simulink model "AUV_SLIDDING_OPTIMAL_2"  (Simulink 7.6)
settings: Solver=ode5  StartTime=0.0  StopTime=200  FixedStep=.1  RelTol=1e-3
libraries: simulink x3
settings Model: Creator=Comp  LastModifiedBy=HP

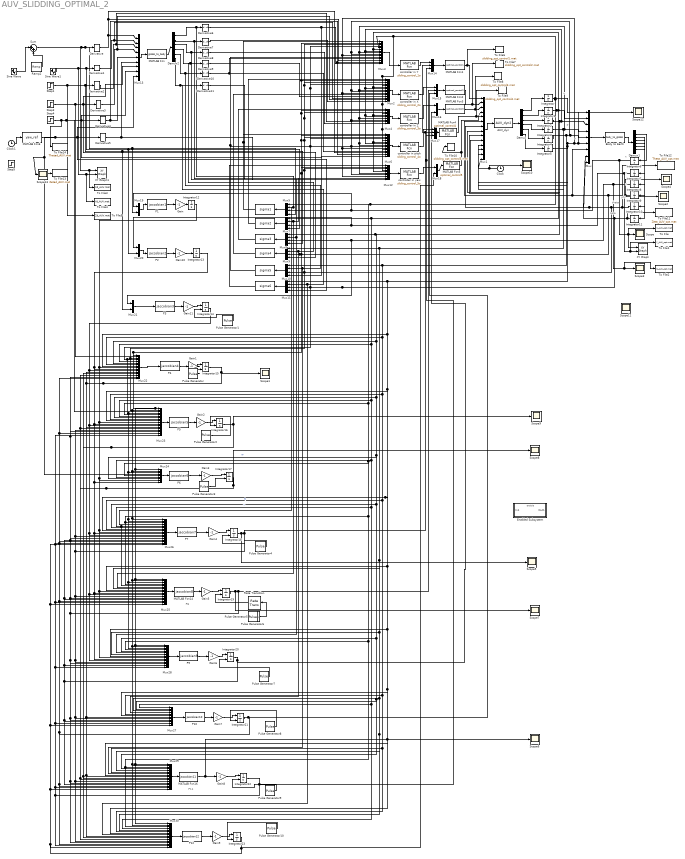
== system AUV_SLIDDING_OPTIMAL_2 ==
  note: u
  note: p
  note: r
  note: x
  note: y
  note: z
  note: phi
  note: theta
  note: zeta
  note: P8
  note: P11
  " " : MATLABFcn  MATLABFcn=sigma6
  "   " : MATLABFcn  MATLABFcn=sigma5
  "    " : MATLABFcn  MATLABFcn=sigma4
  "      " : MATLABFcn  MATLABFcn=sigma3
  "            " : MATLABFcn  MATLABFcn=sigma2
  "                            " : MATLABFcn  MATLABFcn=sigma1
  AUV_dyn : MATLABFcn  MATLABFcn=AUV_dyn2
  Body to Earth : MATLABFcn  MATLABFcn=body_to_global
  Clock : Clock
      settings: Decimation=10
  Clock1 : Clock
  Demux : Demux  Outputs=6
  Demux1 : Demux  Outputs=6
  Demux2 : Demux  Outputs=6
  Derivative{,1..11} (12 alike) : Derivative
  Enabled Subsystem : Subsystem  TreatAsAtomicUnit=on
  Gain{,1..11} (12 alike) : Gain  Gain=-1
  Integrator{,1..6,8..13} (13 alike) : Integrator
  Integrator{14..23} (10 alike) : Integrator  ExternalReset=rising
  Integrator7 : Integrator  InitialCondition=12.5
  MATLAB Fcn : MATLABFcn  MATLABFcn=global_to_body
  MATLAB Fcn1 : MATLABFcn  MATLABFcn=optimal_control1
  MATLAB Fcn14 : MATLABFcn  MATLABFcn=jaccobian8
  MATLAB Fcn16 : MATLABFcn  MATLABFcn=jaccobian11
  MATLAB Fcn2 : MATLABFcn  MATLABFcn=optimal_control2
  MATLAB Fcn3 : MATLABFcn  MATLABFcn=optimal_control3
  MATLAB Fcn4 : MATLABFcn  MATLABFcn=optimal_control4
  MATLAB Fcn5 : MATLABFcn  MATLABFcn=optimal_control5
  MATLAB Fcn6 : MATLABFcn  MATLABFcn=yaw_ref
  Mux : Mux  Inputs=9
  Mux1 : Mux  Inputs=14
  Mux{5,7..11} (6 alike) : Mux
  Mux12 : Mux  Inputs=10
  Mux13 : Mux  Inputs=9
  Mux14 : Mux  Inputs=3
  Mux15 : Mux  Inputs=3
  Mux{16,18..21} (5 alike) : Mux  Inputs=2
  Mux17 : Mux  Inputs=3
  Mux{2..3,6,28} (4 alike) : Mux  Inputs=15
  Mux22 : Mux  Inputs=16
  Mux23 : Mux  Inputs=18
  Mux24 : Mux  Inputs=9
  Mux25 : Mux  Inputs=17
  Mux26 : Mux  Inputs=17
  Mux27 : Mux  Inputs=12
  Mux29 : Mux  Inputs=17
  Mux30 : Mux  Inputs=16
  Mux4 : Mux  Inputs=10
  P1 : MATLABFcn  MATLABFcn=jaccobian1
  P10 : MATLABFcn  MATLABFcn=jaccobian10
  P12 : MATLABFcn  MATLABFcn=jaccobian12
  P2 : MATLABFcn  MATLABFcn=jaccobian2
  P3 : MATLABFcn  MATLABFcn=jaccobian3
  P4 : MATLABFcn  MATLABFcn=jaccobian4
  P5 : MATLABFcn  MATLABFcn=jaccobian5
  P6 : MATLABFcn  MATLABFcn=jaccobian6
  P7 : MATLABFcn  MATLABFcn=jaccobian7
  P9 : MATLABFcn  MATLABFcn=jaccobian9
  Pulse Generator{,1..5,7..10} (10 alike) : DiscretePulseGenerator  PulseType=Time based  Period=1  PulseWidth=50
  Pulse Generator6 : DiscretePulseGenerator
  Ramp2 : simulink/Sources/Ramp  SystemSampleTime=-1  slope=.25  start=0  X0=0
  Rate Transition : RateTransition
  Scope{,1..13} (14 alike) : Scope
      Scope1 settings: YMin=-2e+007  YMax=1.8e+008
      Scope10 settings: YMin=0  YMax=160  SaveName=ScopeData10
      Scope11 settings: SaveName=ScopeData11
      Scope12 settings: YMin=-0.05  YMax=0.6  SaveName=ScopeData12
      Scope13 settings: YMin=0  YMax=250  SaveName=ScopeData13
      Scope2 settings: YMin=-0.08  YMax=0.01  SaveName=ScopeData2
      Scope3 settings: SaveName=ScopeData3
      Scope4 settings: YMin=1  YMax=8.5  SaveName=ScopeData4
      Scope5 settings: YMin=0  YMax=250  SaveName=ScopeData5
      Scope6 settings: SaveName=ScopeData6
      Scope7 settings: YMin=-4.5e+008  YMax=4.5e+008  SaveName=ScopeData7
      Scope8 settings: YMin=-1000  YMax=1750  SaveName=ScopeData8
      Scope9 settings: YMin=-4e+006  YMax=7.5e+006  SaveName=ScopeData9
  Sine Wave : Sin  Amplitude=2.5  Frequency=.1  SampleTime=0
  Sine Wave1 : Sin  Amplitude=12.5  Frequency=.05  Phase=pi/2  SampleTime=0
  Step1 : Step  Time=0  After=5  SampleTime=0
  Step3 : Step  Time=0  After=0  SampleTime=0
  Step4 : Step  Time=0  After=0  SampleTime=0
  Step5 : Step  Time=0  After=0  SampleTime=0
  Sum : Sum  Inputs=|++
  To File : ToFile  Filename=X_AUV_opt.mat  MatrixName=Xo  SaveFormat=Timeseries
  To File1 : ToFile  Filename=Y_AUV_opt.mat  MatrixName=Yo  SaveFormat=Timeseries
  To File10 : ToFile  Filename=slidding_opt_control5.mat  MatrixName=Uo5  SaveFormat=Timeseries
  To File11 : ToFile  Filename=Zeta_AUV_opt.mat  MatrixName=zeta_o  SaveFormat=Timeseries
  To File12 : ToFile  Filename=Theta_AUV_opt.mat  MatrixName=theta_o  SaveFormat=Timeseries
  To File13 : ToFile  Filename=Zetad_AUV.mat  MatrixName=zeta_d  SaveFormat=Timeseries
  To File14 : ToFile  Filename=Thetad_AUV.mat  MatrixName=theta_d  SaveFormat=Timeseries
  To File2 : ToFile  Filename=Z_AUV_opt.mat  MatrixName=Zo  SaveFormat=Timeseries
  To File3 : ToFile  Filename=Xd_AUV.mat  MatrixName=Xd  SaveFormat=Timeseries
  To File4 : ToFile  Filename=Yd_AUV.mat  MatrixName=Yd  SaveFormat=Timeseries
  To File5 : ToFile  Filename=Zd_AUV.mat  MatrixName=Zd  SaveFormat=Timeseries
  To File6 : ToFile  Filename=slidding_opt_control1.mat  MatrixName=Uo1  SaveFormat=Timeseries
  To File7 : ToFile  Filename=slidding_opt_control2.mat  MatrixName=Uo2  SaveFormat=Timeseries
  To File8 : ToFile  Filename=slidding_opt_control3.mat  MatrixName=Uo3  SaveFormat=Timeseries
  To File9 : ToFile  Filename=slidding_opt_control4.mat  MatrixName=Uo4  SaveFormat=Timeseries
  XY Graph : simulink/Sinks/XY Graph  SystemSampleTime=-1  xmin=0  xmax=60  ymin=-20  ymax=20  st=-1
  XY Graph1 : simulink/Sinks/XY Graph  SystemSampleTime=-1  xmin=-20  xmax=20  ymin=-20  ymax=20  st=-1
  controller in X : MATLABFcn  MATLABFcn=sliding_control_2o
  controller in Y : MATLABFcn  MATLABFcn=sliding_control_1o
  controller in Z : MATLABFcn  MATLABFcn=sliding_control_3o
  controller in pitch : MATLABFcn  MATLABFcn=sliding_control_4o
  controller in yaw : MATLABFcn  MATLABFcn=sliding_control_5o
  wires:
  AUV_dyn/1 -> Demux/1
  Demux/1 -> Integrator/1
  Demux/2 -> Integrator1/1
  Demux/3 -> Integrator2/1
  Demux/4 -> Integrator3/1
  Demux/5 -> Integrator4/1
  Demux/6 -> Integrator5/1
  Integrator2/1 -> Mux1/10, Mux/3, Mux3/7, Mux2/7, Mux4/6, Mux6/7, Mux8/1, Mux22/6, Mux23/7, Mux24/7, Mux26/6, Mux28/5, Mux27/2, Mux29/4  "w"
  Integrator4/1 -> Mux1/12, Mux/5, Mux3/9, Mux2/9, Mux4/8, Mux6/9, Mux12/7, Mux10/1, Mux22/7, Mux23/8, Mux26/7, Mux27/5, Mux29/6, Mux30/6  "q"
  Integrator3/1 -> Mux1/11, Mux/4, Mux3/8, Mux2/8, Mux4/7, Mux6/8, Mux12/6, Mux9/1, Mux25/7, Mux28/7, Mux27/3, Mux29/5, Mux30/5
  Mux/1 -> Body to Earth/1
  Integrator/1 -> Mux/1, Mux1/8, Mux3/5, Mux2/5, Mux4/4, Mux6/5, Mux12/4, Mux5/1, Mux23/5, Mux24/5, Mux26/3, Mux25/4, Mux28/4, Mux29/3, Mux30/3
  Integrator1/1 -> Mux/2, Mux1/9, Mux3/6, Mux2/6, Mux4/5, Mux6/6, Mux12/5, Mux7/1, Mux22/5, Mux23/6, Mux24/6, Mux26/5, Mux25/5, Mux27/1, Mux30/4  "v"
  Integrator5/1 -> Mux1/13, Mux3/10, Mux2/10, Mux6/10, Mux12/8, Mux/6, Scope12/1, Mux11/1, Mux22/8, Mux23/9, Mux26/8, Mux25/8, Mux28/8, Mux27/6, Mux29/8, Mux30/7
  Body to Earth/1 -> Demux1/1
  Demux1/1 -> Integrator6/1
  Demux1/2 -> Integrator7/1
  Demux1/3 -> Integrator8/1
  Demux1/4 -> Integrator9/1
  Demux1/5 -> Integrator10/1
  Demux1/6 -> Integrator11/1
  Integrator9/1 -> Mux/7, Mux1/6, Mux3/2, Mux2/2, Mux4/2, Mux6/2, Mux12/2, Mux9/3, Mux22/1, Mux23/1, Mux24/1, Mux25/1, Mux28/1, Mux29/1, Mux30/1, Scope4/1, Scope2/1
  Integrator10/1 -> Mux/8, Mux1/7, Mux10/3, Mux3/3, Mux2/3, Mux4/3, Mux6/3, Mux12/3, Mux22/3, Mux23/2, Mux24/2, Mux26/1, Mux25/2, Mux28/2, Mux29/2, Mux30/2, To File12/1
  Integrator11/1 -> Mux/9, Mux11/3, Mux3/4, Mux2/4, Mux6/4, Mux22/4, Mux23/4, Mux24/3, Mux26/2, Mux25/3, Mux28/3, To File11/1
  Mux5/1 -> "                            "/1
  Integrator6/1 -> Scope/1, XY Graph/1, To File/1, Mux5/3, Mux19/1
  Mux7/1 -> "            "/1
  Integrator7/1 -> XY Graph/2, To File1/1, Mux7/3, Mux20/1
  Mux8/1 -> "      "/1
  Integrator8/1 -> Mux8/3, Mux21/1, Scope3/1, To File2/1
  Mux9/1 -> "    "/1
  Mux10/1 -> "   "/1
  Mux11/1 -> " "/1
  Mux3/1 -> controller in Y/1
  "                            "/1 -> Mux3/1, Mux6/1
  Mux2/1 -> controller in X/1
  Mux4/1 -> controller in Z/1
  Mux6/1 -> controller in pitch/1
  Mux12/1 -> controller in yaw/1
  "   "/1 -> Mux3/11, Mux6/11
  "            "/1 -> Mux2/1
  "    "/1 -> Mux2/11
  "      "/1 -> Mux4/1
  " "/1 -> Mux12/1
  Sum/1 -> Derivative/1, Mux5/4, Mux19/2, XY Graph1/1, To File3/1
  Sine Wave1/1 -> Derivative1/1, Mux7/4, Mux20/2, XY Graph1/2, To File4/1
  Step1/1 -> Derivative2/1, Mux8/4, Mux21/2, To File5/1
  Step3/1 -> Derivative3/1, Mux13/7, Mux9/4, Mux22/2
  Step4/1 -> Derivative4/1, Mux13/8, Mux10/4, Mux23/3, To File14/1
  MATLAB Fcn6/1 -> Derivative5/1, Mux13/9, Mux11/4, Mux24/4, To File13/1, Scope13/1
  Derivative/1 -> Mux13/1, Mux3/13, Mux6/13
  Derivative1/1 -> Mux13/2, Mux2/13
  Derivative2/1 -> Mux13/3, Mux4/9
  Derivative3/1 -> Mux13/4, Mux2/14
  Derivative4/1 -> Mux13/5, Mux3/14, Mux6/14
  Derivative5/1 -> Mux13/6, Mux12/10
  Mux13/1 -> MATLAB Fcn/1
  Demux2/1 -> Derivative6/1, Mux5/2, Mux26/4
  Demux2/2 -> Derivative7/1, Mux7/2, Mux25/6
  Demux2/3 -> Derivative8/1, Mux8/2, Mux28/6
  Demux2/4 -> Derivative9/1, Mux9/2, Mux27/4
  Demux2/5 -> Derivative10/1, Mux10/2, Mux29/7
  Demux2/6 -> Derivative11/1, Mux11/2, Mux30/8
  Derivative10/1 -> Mux3/12, Mux6/12
  Derivative6/1 -> Mux3/15, Mux6/15
  Derivative9/1 -> Mux2/12
  Derivative7/1 -> Mux2/15
  Derivative8/1 -> Mux4/10
  Derivative11/1 -> Mux12/9
  MATLAB Fcn/1 -> Demux2/1
  MATLAB Fcn1/1 -> Mux1/1, To File6/1
  controller in Y/1 -> Mux14/1
  Mux14/1 -> MATLAB Fcn1/1
  Mux15/1 -> MATLAB Fcn2/1
  MATLAB Fcn2/1 -> Mux1/2, To File7/1
  controller in X/1 -> Mux15/1
  Mux16/1 -> MATLAB Fcn3/1
  MATLAB Fcn3/1 -> Mux1/3, To File8/1
  controller in Z/1 -> Mux16/1
  MATLAB Fcn4/1 -> Mux1/4, To File9/1
  Mux17/1 -> MATLAB Fcn4/1
  controller in pitch/1 -> Mux17/1
  MATLAB Fcn5/1 -> Mux1/5, To File10/1
  Mux18/1 -> MATLAB Fcn5/1
  controller in yaw/1 -> Mux18/1
  Mux19/1 -> P1/1
  Mux20/1 -> P2/1
  Mux21/1 -> P3/1
  Mux22/1 -> P4/1
  Integrator12/1 -> Mux22/9, Mux23/10, Mux24/8, Mux26/9, Mux25/9, Mux28/9
  Integrator13/1 -> Mux22/10, Mux23/11, Mux24/9, Mux26/10, Mux25/10, Mux28/10
  Integrator14/1 -> Mux22/11, Mux23/12, Mux26/11, Mux25/11, Mux28/11
  Integrator15/1 -> Mux22/12, Mux23/13, Mux27/7, Mux29/9, Mux30/9, Scope1/1
  Integrator16/1 -> Mux22/13, Mux29/10, Mux30/10, Scope9/1
  Integrator17/1 -> Mux22/14, Mux23/14, Mux29/11, Mux30/11, Scope8/1
  Integrator19/1 -> Mux22/15, Mux23/16, Mux26/13, Mux25/13, Mux28/13, Mux27/9, Mux29/13, Mux30/13, Mux15/2, Scope7/1
  Integrator21/1 -> Mux22/16, Mux23/17, Mux26/15, Mux25/15, Mux29/15, Mux30/14, Mux15/3
  Integrator18/1 -> Mux23/15, Mux26/12, Mux25/12, Mux28/12, Mux27/8, Mux29/12, Mux30/12, Mux14/2, Mux17/2, Scope5/1
  Integrator22/1 -> Mux23/18, Mux26/16, Mux25/16, Mux28/15, Mux27/11, Mux29/16, Mux30/15, Mux14/3, Mux17/3
  Mux24/1 -> P6/1
  Mux26/1 -> P7/1
  Integrator20/1 -> Mux26/14, Mux25/14, Mux28/14, Mux27/10, Mux29/14, Mux16/2
  Integrator23/1 -> Mux26/17, Mux25/17, Mux27/12, Mux29/17, Mux30/16, Mux18/2
  Mux25/1 -> MATLAB Fcn14/1
  Mux23/1 -> P5/1
  Mux28/1 -> P9/1
  Mux27/1 -> P10/1
  Mux30/1 -> P12/1
  Mux29/1 -> MATLAB Fcn16/1
  Mux1/1 -> AUV_dyn/1
  P1/1 -> Gain/1
  Gain/1 -> Integrator12/1
  P6/1 -> Gain3/1
  Gain3/1 -> Integrator17/1
  P7/1 -> Gain4/1
  Gain4/1 -> Integrator18/1
  MATLAB Fcn14/1 -> Gain5/1
  Gain5/1 -> Integrator19/1
  P9/1 -> Gain6/1
  Gain6/1 -> Integrator20/1
  P10/1 -> Gain7/1
  Gain7/1 -> Integrator21/1
  MATLAB Fcn16/1 -> Gain8/1, Scope6/1
  Gain8/1 -> Integrator22/1
  P12/1 -> Gain9/1
  Gain9/1 -> Integrator23/1
  P5/1 -> Gain2/1
  Gain2/1 -> Integrator16/1
  P4/1 -> Gain1/1
  Gain1/1 -> Integrator15/1
  P2/1 -> Gain10/1
  Gain10/1 -> Integrator13/1
  P3/1 -> Gain11/1
  Gain11/1 -> Integrator14/1
  Clock/1 -> Mux1/14, Scope10/1
  Sine Wave/1 -> Sum/1
  Pulse Generator/1 -> Integrator15/2
  Pulse Generator1/1 -> Integrator14/2
  Pulse Generator2/1 -> Integrator16/2
  Pulse Generator3/1 -> Integrator17/2
  Pulse Generator4/1 -> Integrator18/2
  Pulse Generator7/1 -> Integrator20/2
  Pulse Generator8/1 -> Integrator21/2
  Pulse Generator9/1 -> Integrator22/2
  Pulse Generator10/1 -> Integrator23/2
  Pulse Generator5/1 -> Rate Transition/1
  Rate Transition/1 -> Integrator19/2
  Ramp2/1 -> Sum/2
  Clock1/1 -> MATLAB Fcn6/1

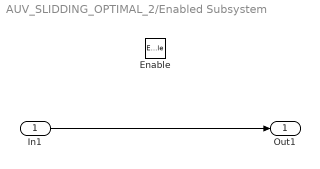
== system AUV_SLIDDING_OPTIMAL_2/Enabled Subsystem ==
  In1 : Inport
  Enable : EnablePort
  Out1 : Outport
  wires:
  In1/1 -> Out1/1
